simulink model "Benchmark11APR24"  (R2023b)
settings: Solver=VariableStepAuto  StartTime=0.0  StopTime=10  RelTol=1e-3
settings Model: Creator=Joseph Mockler  LastModifiedBy=Joseph Mockler

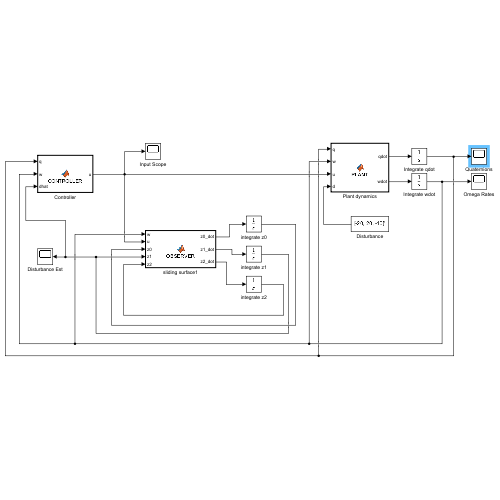
[thumbnail: Simulink's stored preview of the top-level diagram]
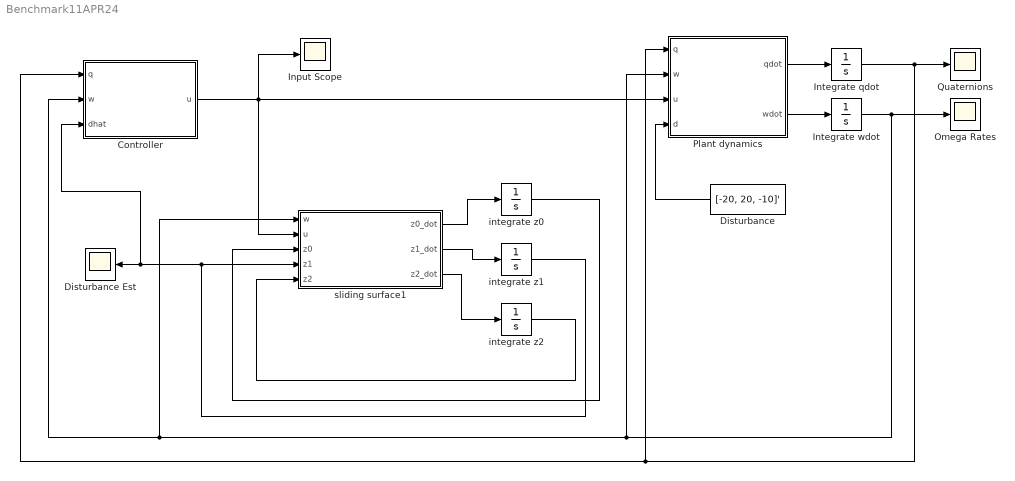
== system Benchmark11APR24 ==
  Controller : MATLAB Function  TreatAsAtomicUnit=on
  Disturbance : Constant  Value=[-20, 20, -10]'
  Disturbance Est : Scope
  Input Scope : Scope
  Integrate qdot : Integrator  InitialCondition=[0.081, 0.054, 0.126, 0]'
  Integrate wdot : Integrator
  Omega Rates : Scope
  Plant dynamics : MATLAB Function  TreatAsAtomicUnit=on
  Quaternions : Scope
  integrate z0 : Integrator
  integrate z1 : Integrator
  integrate z2 : Integrator
  sliding surface1 : MATLAB Function  TreatAsAtomicUnit=on
  wires:
  Plant dynamics/1(qdot) -> Integrate qdot/1
  Plant dynamics/2(wdot) -> Integrate wdot/1
  Disturbance/1 -> Plant dynamics/4(d)
  sliding surface1/1(z0_dot) -> integrate z0/1
  Integrate wdot/1 -> Omega Rates/1, Controller/2(w), sliding surface1/1(w), Plant dynamics/2(w)
  sliding surface1/2(z1_dot) -> integrate z1/1
  sliding surface1/3(z2_dot) -> integrate z2/1
  Integrate qdot/1 -> Quaternions/1, Controller/1(q), Plant dynamics/1(q)
  integrate z2/1 -> sliding surface1/5(z2)
  integrate z0/1 -> sliding surface1/3(z0)
  integrate z1/1 -> Controller/3(dhat), Disturbance Est/1, sliding surface1/4(z1)
  Controller/1(u) -> Plant dynamics/3(u), Input Scope/1, sliding surface1/2(u)

== matlab function Benchmark11APR24/Controller ==
  data: q input; w input; u output; dhat input
function u = CONTROLLER(q, w, dhat)

u = [0;0;0];

%C1 = (Ixz)/(Ixx*Izz-Ixz^2);
%C2 = (Ixx)/(Ixx*Izz-Ixz^2);
%C3 = 1/Iyy;
%C4 = (Izz)/(Ixx*Izz-Ixz^2);


%A = [C4*Lp, 0, C1*Nr;
%    0, C3*Mq, 0;
%    Cq*Lp, 0, C2*Nr];
%B = [C4*Ldp, C1*Ndb, 0;
%    0, 0, C3*Mp;
%    C1*Ldp, C2*Ndb, 0];

A = [-15.20, 0, -19.31;
    0, -2.61, 0;
    -8.13, 0, -43.18];

B = [4275.35, 2860.64, 0;
    0, 0, 3590.66;
    2288.51, 6397.42, 0];

q1 = q(1);
q2 = q(2);
q3 = q(3);
q4 = q(4);

T = [q4, -q3, q2;
    q3, q4, -q1;
    -q2, q1, q4];

zeta = 0.01;
G = 20*eye(3);
k1 = 20;
k2 = 500;
s = w + G*[q1, q2, q3]';
mag_s = sqrt(s'*s);

s_sigma = [abs(s(1))^(0.8)*sign(s(1));
        abs(s(2))^(0.8)*sign(s(2))
        abs(s(3))^(0.8)*sign(s(3))];

u = -inv(B)*((A*w + 0.5*G*T*w) + dhat + k1*s + k2*s*(1/(mag_s^0.8+zeta)));
%u = -inv(B)*((A*w + 0.5*G*T*w) + dhat + k1*s + k2*s_sigma);

== matlab function Benchmark11APR24/Plant dynamics ==
  data: q input; w input; qdot output; u input; d input; wdot output
function [qdot, wdot] = PLANT(q, w, u, d)

qdot = [0;0;0;0];
wdot = [0;0;0];

%C1 = (Ixz)/(Ixx*Izz-Ixz^2);
%C2 = (Ixx)/(Ixx*Izz-Ixz^2);
%C3 = 1/Iyy;
%C4 = (Izz)/(Ixx*Izz-Ixz^2);


%A = [C4*Lp, 0, C1*Nr;
%    0, C3*Mq, 0;
%    Cq*Lp, 0, C2*Nr];
%B = [C4*Ldp, C1*Ndb, 0;
%    0, 0, C3*Mp;
%    C1*Ldp, C2*Ndb, 0];

A = [-15.20, 0, -19.31;
    0, -2.61, 0;
    -8.13, 0, -43.18];

B = [4275.35, 2860.64, 0;
    0, 0, 3590.66;
    2288.51, 6397.42, 0];

q1 = q(1);
q2 = q(2);
q3 = q(3);
q4 = q(4);

T = [q4, -q3, q2;
    q3, q4, -q1;
    -q2, q1, q4];

qdot_13 = 0.5*T*w;
qdot_4 = -0.5*[q1, q2, q3]*w;
qdot = [qdot_13; qdot_4];
wdot = A*w + B*u + d;

== matlab function Benchmark11APR24/sliding surface1 ==
  data: w input; u input; z0 input; z1 input; z0_dot output; z2 input; z1_dot output; z2_dot output
function [z0_dot, z1_dot, z2_dot] = OBSERVER(w, u, z0, z1, z2)

z0_dot = [0;0;0];
z1_dot = [0;0;0];
z2_dot = [0;0;0];

A = [-15.20, 0, -19.31;
    0, -2.61, 0;
    -8.13, 0, -43.18];

B = [4275.35, 2860.64, 0;
    0, 0, 3590.66;
    2288.51, 6397.42, 0];

L = 1000;
L0 = L^(1/3)*eye(3);
L1 = L^(2/3)*eye(3);
L2 = L^(0)*eye(3);

lambda0 = 3;
lambda1 = 1.5*sqrt(3);
lambda2 = 1.1;
n = 2;

error = z0-w;

sigma0 = [abs(error(1))^(2/3)*sign(error(1));
        abs(error(2))^(2/3)*sign(error(2))
        abs(error(3))^(2/3)*sign(error(3))];

sigma1 = [abs(error(1))^(1/3)*sign(error(1));
        abs(error(2))^(1/3)*sign(error(2))
        abs(error(3))^(1/3)*sign(error(3))];

sigma2 = [abs(error(1))^(0)*sign(error(1));
        abs(error(2))^(0)*sign(error(2))
        abs(error(3))^(0)*sign(error(3))];

z0_dot = -lambda2*L0*(sigma0) + A*w + B*u + z1;
z1_dot = -lambda1*L1*(sigma1) + z2;
z2_dot = -lambda0*L2*(sigma2);
